simulink model "robot2D_2018"  (Simulink 9.2)
settings: Solver=FixedStepAuto  StartTime=0.0  StopTime=10.0  FixedStep=0.001  RelTol=1e-3
values from neighbouring files (symbols this model uses):
  K = place(A, B, [-5 -5 -4 -4])    [script.m]
  Ki = 0.5    [script.m]
settings Model: Creator=alexa  LastModifiedBy=UTCN-C12
settings DataIOCC: LimitDataPoints=off  SaveFormat=Dataset  SignalLoggingSaveFormat=Dataset  ReturnWorkspaceOutputs=on
settings OptimizationCC: LifeSpan=auto
settings DebuggingCC: UnderspecifiedInitializationDetection=Simplified  MergeDetectMultiDrivingBlocksExec=error  FcnCallInpInsideContextMsg=error  UnconnectedInputMsg=none  UnconnectedOutputMsg=none  UnconnectedLineMsg=none  StateNameClashWarn=none  SFUnexpectedBacktrackingDiag=error  SFNoUnconditionalDefaultTransitionDiag=error  SFExecutionAtInitializationDiag=warning  SFMachineParentedDataDiag=error
settings HardwareCC: ProdBitPerPointer=64  ProdBitPerSizeT=64  ProdBitPerPtrDiffT=64  ProdLargestAtomicFloat=Float  ProdIntDivRoundTo=Zero  ProdEndianess=LittleEndian  ProdWordSize=64  ProdHWDeviceType=Intel->x86-64 (Windows64)
settings ModelReferenceCC: PropagateSignalLabelsOutOfModel=on
settings SFSimCC: SimUseLocalCustomCode=on
settings RTWCC: RTWUseLocalCustomCode=on
settings CodeAppCC: StateflowObjectComments=off
settings GRTTargetCC: TargetLangStandard=C99 (ISO)  GeneratePreprocessorConditionals=Use local settings  CombineOutputUpdateFcns=on  GRTInterface=off
settings ConfigComp: CovMetricSettings=dwe  CovHtmlReporting=off  CovSaveCumulativeToWorkspaceVar=off  CovSaveSingleToWorkspaceVar=off  CovExternalEMLEnable=on

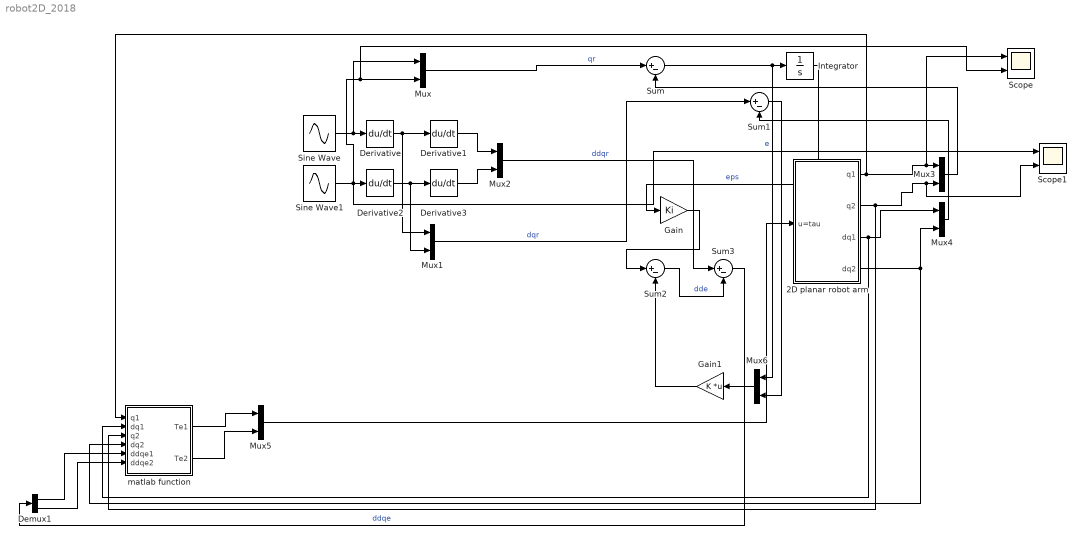
== system robot2D_2018 ==
  2D planar robot arm : Subsystem
  Demux1 : Demux  Outputs=2
  Derivative{,1..3} (4 alike) : Derivative
  Gain : Gain  Gain=Ki
  Gain1 : Gain  Gain=K  Multiplication=Matrix(K*u)
  Integrator : Integrator
  Mux{,1..6} (7 alike) : Mux  Inputs=2
  Scope : Scope  NumInputPorts=2
  Scope1 : Scope  NumInputPorts=2
  Sine Wave : Sin  SampleTime=0
  Sine Wave1 : Sin  SampleTime=0
  Sum{,1..3} (4 alike) : Sum  Inputs=|+-
  matlab function : MATLAB Function  TreatAsAtomicUnit=on
  wires:
  Sine Wave/1 -> Mux/1, Derivative/1
  Derivative/1 -> Mux1/1, Derivative1/1
  Derivative2/1 -> Mux1/2, Derivative3/1
  Sine Wave1/1 -> Scope/2, Mux/2, Derivative2/1, Scope1/1
  Derivative1/1 -> Mux2/1
  Derivative3/1 -> Mux2/2
  2D planar robot arm/1(q1) -> matlab function/1(q1), Scope/1, Mux3/1
  2D planar robot arm/2(q2) -> matlab function/3(q2), Scope1/2, Mux3/2
  2D planar robot arm/3(dq1) -> matlab function/2(dq1), Mux4/1
  2D planar robot arm/4(dq2) -> matlab function/4(dq2), Mux4/2
  Mux/1 -> Sum/1  "qr"
  Mux3/1 -> Sum/2
  Mux1/1 -> Sum1/1  "dqr"
  Mux4/1 -> Sum1/2
  Sum/1 -> Mux6/1, Integrator/1  "e"
  Integrator/1 -> Gain/1  "eps"
  Sum1/1 -> Mux6/2
  Mux6/1 -> Gain1/1
  Gain/1 -> Sum2/1
  Gain1/1 -> Sum2/2
  Mux2/1 -> Sum3/1  "ddqr"
  Sum2/1 -> Sum3/2  "dde"
  Demux1/2 -> matlab function/6(ddqe2)
  Demux1/1 -> matlab function/5(ddqe1)
  matlab function/2(Te2) -> Mux5/2
  matlab function/1(Te1) -> Mux5/1
  Mux5/1 -> 2D planar robot arm/1(u=tau)
  Sum3/1 -> Demux1/1  "ddqe"

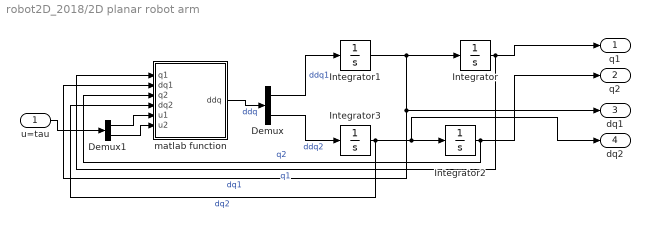
== system robot2D_2018/2D planar robot arm ==
  u=tau : Inport
  Demux : Demux  Outputs=2
  Demux1 : Demux  Outputs=2
  Integrator{,1..3} (4 alike) : Integrator
  matlab function : MATLAB Function  TreatAsAtomicUnit=on
  q1 : Outport  VectorParamsAs1DForOutWhenUnconnected=on
  q2 : Outport  Port=2  VectorParamsAs1DForOutWhenUnconnected=on
  dq1 : Outport  Port=3  VectorParamsAs1DForOutWhenUnconnected=on
  dq2 : Outport  Port=4  VectorParamsAs1DForOutWhenUnconnected=on
  wires:
  Demux1/1 -> matlab function/5(u1)
  Integrator1/1 -> matlab function/2(dq1), dq1/1, Integrator/1  "dq1"
  Demux/2 -> Integrator3/1  "ddq2"
  Integrator2/1 -> matlab function/3(q2), q2/1  "q2"
  Integrator3/1 -> matlab function/4(dq2), dq2/1, Integrator2/1  "dq2"
  matlab function/1(ddq) -> Demux/1  "ddq"
  Demux1/2 -> matlab function/6(u2)
  Demux/1 -> Integrator1/1  "ddq1"
  Integrator/1 -> matlab function/1(q1), q1/1  "q1"
  u=tau/1 -> Demux1/1

== matlab function 2D planar robot arm/matlab function ==
  data: q1 input double; ddq output double; dq1 input double; q2 input double; dq2 input double; u1 input double; u2 input double
function ddq = fcn(q1,dq1,q2,dq2,u1,u2)

D=[0.003515*cos(q2)+0.000925*cos(q2)^2+0.026254,      0
                                               0, 0.023625];

C=[0.24-0.5*dq2*(0.000925*sin(2.0*q2)+0.003515*sin(q2)), -0.004625*dq1*(0.1*sin(2.0*q2)+0.38*sin(q2))
    0.004625*dq1*(0.1*sin(2.0*q2)+0.38*sin(q2)),                0.16];

G = [-4.905*sin(q1)*(0.037*cos(q2)+0.079325)
                 -0.18149*cos(q1)*sin(q2)];

ddq=inv(D)*(-C*[dq1;dq2]-G+[u1;u2]);

== matlab function matlab function ==
  data: q1 input double; Te1 output double; dq1 input double; q2 input double; dq2 input double; ddqe1 input double; ddqe2 input double; Te2 output double
function [Te1, Te2] = fcn(q1,dq1,q2,dq2,ddqe1,ddqe2)

D=[0.003515*cos(q2)+0.000925*cos(q2)^2+0.026254,      0
                                               0, 0.023625];

C=[0.24-0.5*dq2*(0.000925*sin(2.0*q2)+0.003515*sin(q2)), -0.004625*dq1*(0.1*sin(2.0*q2)+0.38*sin(q2))
    0.004625*dq1*(0.1*sin(2.0*q2)+0.38*sin(q2)),                0.16];

G = [-4.905*sin(q1)*(0.037*cos(q2)+0.079325)
                 -0.18149*cos(q1)*sin(q2)];


Te = D*[ddqe1; ddqe2] + C * [dq1;dq2] + G;

Te1 = Te(1);
Te2 = Te(2);
